simulink model "discsim"  (Simulink 8.0)
settings: Solver=ode3  StartTime=0.0  StopTime=10000  FixedStep=ts  RelTol=1e-3
values from neighbouring files (symbols this model uses):
  sysD = c2d(sys,ts)    [contsimu.m]    (also in disc2.m; discreteship.m; test2.m = ss(A,B,C,0,ts))
  sysD_F = lqr(sysD,Q,R)    [contsimu.m]
  sysD_N = Nufd + sysD_F*Nxfd    [contsimu.m]
  ts = 0.01    [aaushipcode.m]    (also in contsimu.m = 1; disc2.m; discreteship.m; kalman.m = 0.1)
libraries: simulink x1
settings Model: Creator=Lunde  LastModifiedBy=Lunde
settings DataIOCC: SignalLoggingSaveFormat=ModelDataLogs
settings DebuggingCC: FcnCallInpInsideContextMsg=EnableAllAsWarning

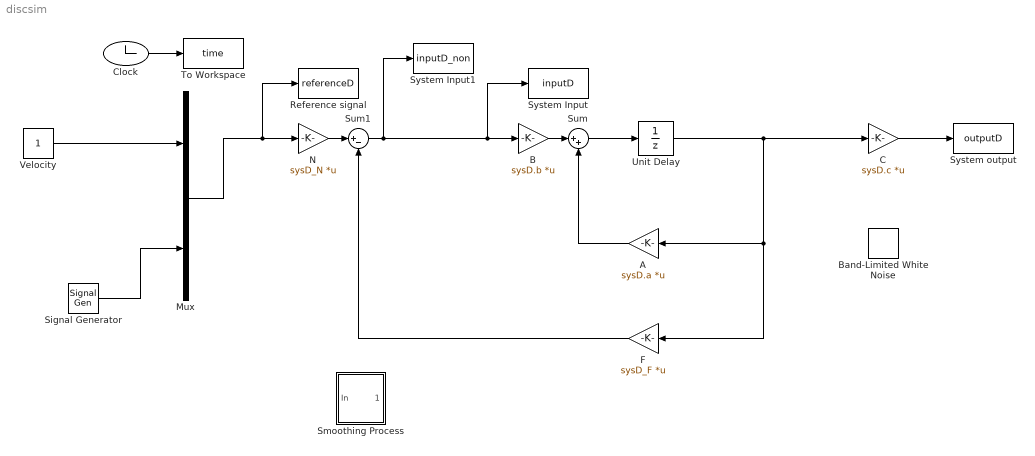
== system discsim ==
  A : Gain  Gain=sysD.a  Multiplication=Matrix(K*u)
  B : Gain  Gain=sysD.b  Multiplication=Matrix(K*u)
  Band-Limited White Noise : simulink/Sources/Band-Limited White Noise  Cov=[0.00001]  Ts=ts  seed=[23341]
  C : Gain  Gain=sysD.c  Multiplication=Matrix(K*u)
  Clock : Clock
  F : Gain  Gain=sysD_F  Multiplication=Matrix(K*u)
  Mux : Mux  Inputs=2
  N : Gain  Gain=sysD_N  Multiplication=Matrix(K*u)  SampleTime=ts
  Reference signal : ToWorkspace  VariableName=referenceD  SampleTime=ts
  Signal Generator : SignalGenerator  WaveForm=sawtooth  Amplitude=pi/2  Frequency=0.001
  Smoothing Process : Subsystem
  Sum : Sum  Inputs=|++
  Sum1 : Sum  Inputs=|+-
  System Input : ToWorkspace  VariableName=inputD  SampleTime=-1
  System Input1 : ToWorkspace  VariableName=inputD_non  SampleTime=-1
  System output : ToWorkspace  VariableName=outputD  SampleTime=-1
  To Workspace : ToWorkspace  VariableName=time  SampleTime=-1
  Unit Delay : UnitDelay  SampleTime=-1
  Velocity : Constant
  wires:
  A/1 -> Sum/2
  B/1 -> Sum/1
  Sum/1 -> Unit Delay/1
  Sum1/1 -> System Input/1, B/1, System Input1/1
  N/1 -> Sum1/1
  Velocity/1 -> Mux/1
  C/1 -> System output/1
  Clock/1 -> To Workspace/1
  F/1 -> Sum1/2
  Mux/1 -> Reference signal/1, N/1
  Unit Delay/1 -> A/1, F/1, C/1
  Signal Generator/1 -> Mux/2

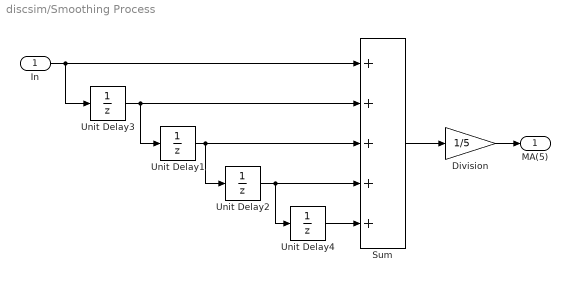
== system discsim/Smoothing Process ==
  In : Inport
  Division : Gain  Gain=1/5
  Sum : Sum  Inputs=+++++
  Unit Delay{1..4} (4 alike) : UnitDelay  SampleTime=-1
  MA(5) : Outport
  wires:
  In/1 -> Unit Delay3/1, Sum/1
  Unit Delay3/1 -> Unit Delay1/1, Sum/2
  Unit Delay1/1 -> Sum/3, Unit Delay2/1
  Unit Delay2/1 -> Sum/4, Unit Delay4/1
  Unit Delay4/1 -> Sum/5
  Sum/1 -> Division/1
  Division/1 -> MA(5)/1
